simulink model "gyroscope_sym"  (R2025b)
settings: Solver=VariableStepAuto  StartTime=0.0  StopTime=10.0  RelTol=1e-3
values from neighbouring files (symbols this model uses):
  A_bn0 = eye(3)    [gyroscope.m]
  D_bias_inst = 0.3/3600    (= 8.33333333333e-05)    [gyroscope.m]
  D_RW = RRW/sqrt(3600)    [gyroscope.m]
  D_wn = D_ARW/sqrt(3600)    [gyroscope.m]
  I = diag([Ix Iy Iz])    [gyroscope.m]
  O = [1,      eps_xy, eps_xz ... (first row only)    [gyroscope.m]
  run_run_bias = 4/3600    (= 0.00111111111111)    [gyroscope.m]
  SFE = 500*1e-6    (= 0.0005)    [gyroscope.m]
  SFN = 15*1e-6    (= 1.5e-05)    [gyroscope.m]
  static_temp_bias = 9/3600    (= 0.0025)    [gyroscope.m]
  theta_eps = [0,            -theta_eps_z,  theta_eps_y ... (first row only)    [gyroscope.m]
  Ts = 1/update_rate    (= 0.01)    [gyroscope.m]
  w0 = [1e-6; 1e-6; n]    [gyroscope.m]
undefined symbols (not defined in the file or in its folder): DiscIntNeverNeededParam
libraries: matrix_library x4, simulink_extras x1
settings Model: Creator=filip  LastModifiedBy=nicol

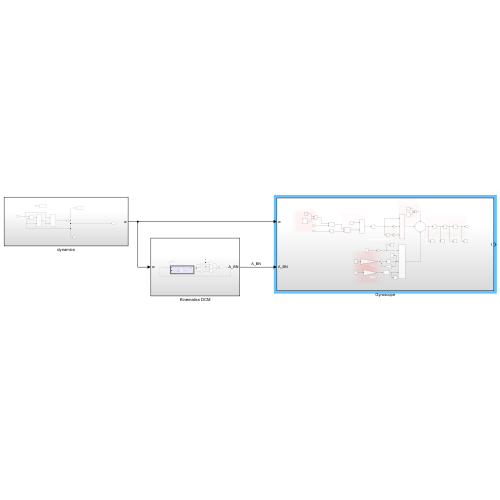
[thumbnail: Simulink's stored preview of the top-level diagram]
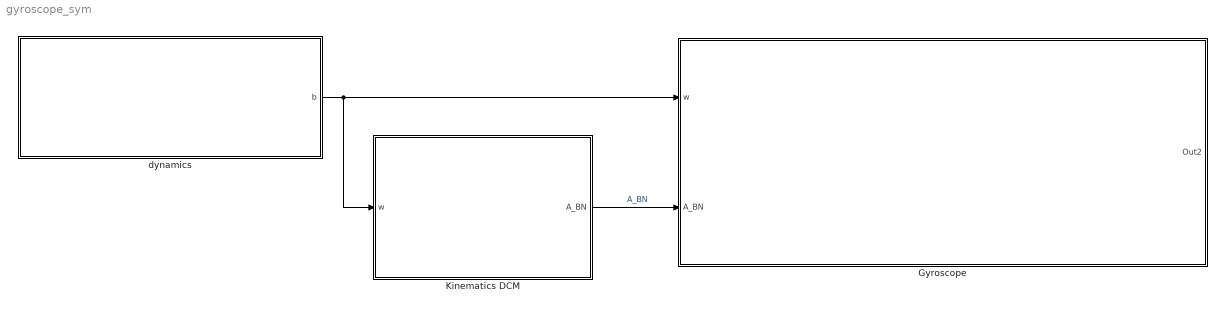
== system gyroscope_sym ==
  Gyroscope : Subsystem
  Kinematics DCM : Subsystem
  dynamics : Subsystem
  wires:
  dynamics/1(b) -> Gyroscope/1(w), Kinematics DCM/1(w)
  Kinematics DCM/1(A_BN) -> Gyroscope/2(A_BN)  "A_BN"

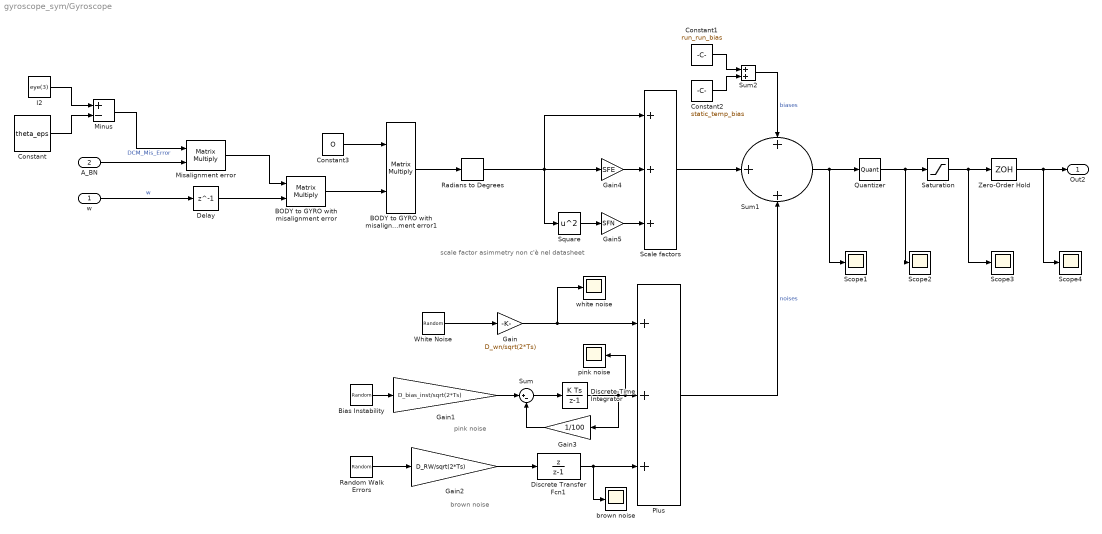
== system gyroscope_sym/Gyroscope ==
  note: scale factor asimmetry non c'è nel datasheet
  note: pink noise
  note: brown noise
  w : Inport
  A_BN : Inport  Port=2
  " White Noise" : RandomNumber  SampleTime=0.1
  BODY to GYRO with misalignment error : Product  Multiplication=Matrix(*)
  BODY to GYRO with misalignment error1 : Product  Multiplication=Matrix(*)
  Bias Instability : RandomNumber  SampleTime=0.1
  Constant : Constant  Value=theta_eps
  Constant1 : Constant  Value=run_run_bias
  Constant2 : Constant  Value=static_temp_bias
  Constant3 : Constant  Value=O
  Delay : Delay  DelayLength=1
  Discrete Transfer Fcn1 : DiscreteTransferFcn  Numerator=[1 0]  Denominator=[1 -1]
  Discrete-Time Integrator : DiscreteIntegrator  ICPrevOutput=DiscIntNeverNeededParam  ICPrevScaledInput=DiscIntNeverNeededParam
  Gain : Gain  Gain=D_wn/sqrt(2*Ts)
  Gain1 : Gain  Gain=D_bias_inst/sqrt(2*Ts)
  Gain2 : Gain  Gain=D_RW/sqrt(2*Ts)
  Gain3 : Gain  Gain=1/100
  Gain4 : Gain  Gain=SFE
  Gain5 : Gain  Gain=SFN
  I2 : Constant  Value=eye(3)
  Minus : Sum  Inputs=+-
  Misalignment error : Product  Multiplication=Matrix(*)
  Plus : Sum  Inputs=+++
  Quantizer : Quantizer  QuantizationInterval=LSB
  Radians to Degrees : simulink_extras/Transformations/Radians to Degrees
  Random Walk Errors : RandomNumber  SampleTime=0.1
  Saturation : Saturate  UpperLimit=20  LowerLimit=-20
  Scale factors : Sum  Inputs=+++
  Scope{1..4} (4 alike) : Scope
      Scope1 settings: ActiveDisplayYMinimum=-0.032120647567430112  ActiveDisplayYMaximum=0.096644162809020939  DataLoggingVariableName=ScopeData2
      Scope2 settings: ActiveDisplayYMinimum=-1  ActiveDisplayYMaximum=1  DataLoggingVariableName=ScopeData3
      Scope3 settings: ActiveDisplayYMinimum=-1  ActiveDisplayYMaximum=1  DataLoggingVariableName=ScopeData4
      Scope4 settings: ActiveDisplayYMinimum=-0.032120647471039  ActiveDisplayYMaximum=0.096644162883216228  DataLoggingVariableName=ScopeData5
  Square : Math  Operator=square
  Sum : Sum  Inputs=|+-
  Sum1 : Sum  Inputs=+++
  Sum2 : Sum
  Zero-Order Hold : ZeroOrderHold  SampleTime=Ts
  brown noise : Scope
      settings: ActiveDisplayYMinimum=-0.025691906984189852  ActiveDisplayYMaximum=0.0025755592198982418  DataLoggingVariableName=ScopeData10
  pink noise : Scope
      settings: ActiveDisplayYMinimum=-0.013777619312277414  ActiveDisplayYMaximum=0.014220901201123974  DataLoggingVariableName=ScopeData9
  white noise : Scope
      settings: ActiveDisplayYMinimum=-0.0017013348354620785  ActiveDisplayYMaximum=0.001720930099973718  DataLoggingVariableName=ScopeData8
  Out2 : Outport
  wires:
  Sum1/1 -> Scope1/1, Quantizer/1
  Gain1/1 -> Sum/1
  A_BN/1 -> Misalignment error/2
  Discrete-Time Integrator/1 -> pink noise/1, Plus/2, Gain3/1
  Gain/1 -> white noise/1, Plus/1
  Plus/1 -> Sum1/3  "noises"
  Random Walk Errors/1 -> Gain2/1
  Constant1/1 -> Sum2/1
  Bias Instability/1 -> Gain1/1
  Discrete Transfer Fcn1/1 -> Plus/3, brown noise/1
  Sum/1 -> Discrete-Time Integrator/1
  I2/1 -> Minus/1
  " White Noise"/1 -> Gain/1
  w/1 -> Delay/1  "w"
  Quantizer/1 -> Scope2/1, Saturation/1
  Minus/1 -> Misalignment error/1  "DCM_Mis_Error"
  Misalignment error/1 -> BODY to GYRO with misalignment error/1
  Saturation/1 -> Scope3/1, Zero-Order Hold/1
  Gain3/1 -> Sum/2
  Zero-Order Hold/1 -> Scope4/1, Out2/1
  Gain2/1 -> Discrete Transfer Fcn1/1
  Delay/1 -> BODY to GYRO with misalignment error/2
  BODY to GYRO with misalignment error/1 -> BODY to GYRO with misalignment error1/2
  Radians to Degrees/1 -> Scale factors/1, Gain4/1, Square/1
  Gain4/1 -> Scale factors/2
  Scale factors/1 -> Sum1/2
  Constant2/1 -> Sum2/2
  Sum2/1 -> Sum1/1  "biases"
  Constant/1 -> Minus/2
  Square/1 -> Gain5/1
  Gain5/1 -> Scale factors/3
  Constant3/1 -> BODY to GYRO with misalignment error1/1
  BODY to GYRO with misalignment error1/1 -> Radians to Degrees/1

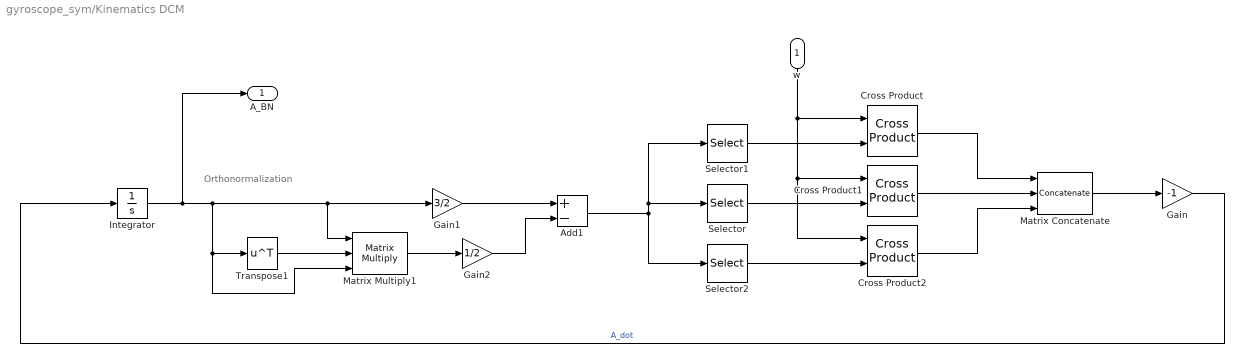
== system gyroscope_sym/Kinematics DCM ==
  note: Orthonormalization
  w : Inport
  Add1 : Sum  Inputs=+-
  Cross Product : matrix_library/Cross Product
  Cross Product1 : matrix_library/Cross Product
  Cross Product2 : matrix_library/Cross Product
  Gain : Gain  Gain=-1
  Gain1 : Gain  Gain=3/2
  Gain2 : Gain  Gain=1/2
  Integrator : Integrator  InitialCondition=A_bn0
  Matrix Concatenate : Concatenate  NumInputs=3  Mode=Multidimensional array  ConcatenateDimension=2
  Matrix Multiply1 : Product  Inputs=3  Multiplication=Matrix(*)
  Selector : Selector  NumberOfDimensions=2  InputPortWidth=3  IndexOptions=Select all,Index vector (dialog)  Indices=[1 3],2  OutputSizes=1,1
  Selector1 : Selector  NumberOfDimensions=2  InputPortWidth=3  IndexOptions=Select all,Index vector (dialog)  Indices=[1 3],1  OutputSizes=1,1
  Selector2 : Selector  NumberOfDimensions=2  InputPortWidth=3  IndexOptions=Select all,Index vector (dialog)  Indices=[1 3],3  OutputSizes=1,1
  Transpose1 : Math  Operator=transpose
  A_BN : Outport
  wires:
  Transpose1/1 -> Matrix Multiply1/2
  w/1 -> Cross Product/1, Cross Product1/1, Cross Product2/1
  Gain/1 -> Integrator/1  "A_dot"
  Gain2/1 -> Add1/2
  Selector/1 -> Cross Product1/2
  Cross Product2/1 -> Matrix Concatenate/3
  Cross Product1/1 -> Matrix Concatenate/2
  Matrix Concatenate/1 -> Gain/1
  Selector1/1 -> Cross Product/2
  Add1/1 -> Selector/1, Selector1/1, Selector2/1
  Matrix Multiply1/1 -> Gain2/1
  Selector2/1 -> Cross Product2/2
  Integrator/1 -> A_BN/1, Transpose1/1, Matrix Multiply1/3, Gain1/1, Matrix Multiply1/1
  Cross Product/1 -> Matrix Concatenate/1
  Gain1/1 -> Add1/1

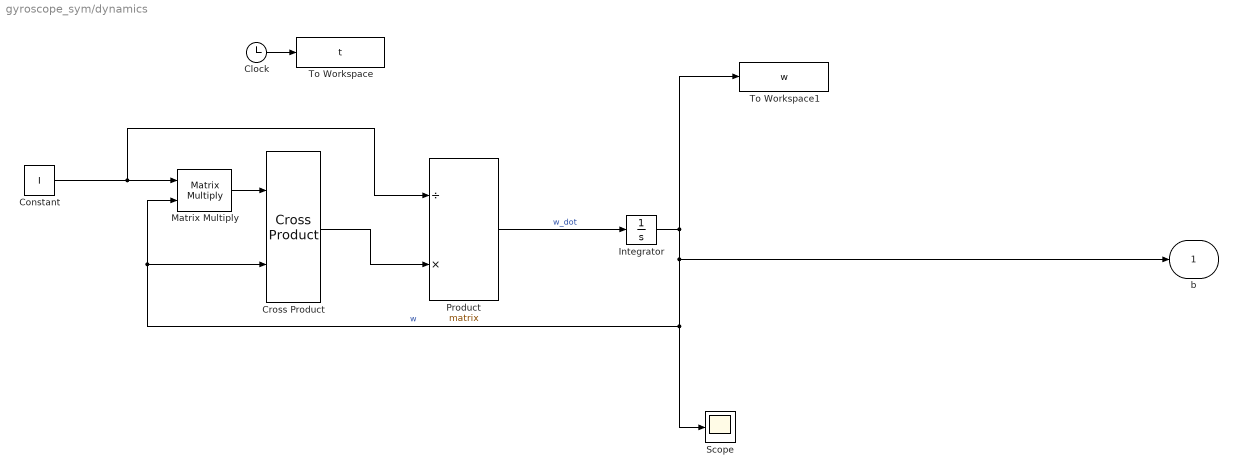
== system gyroscope_sym/dynamics ==
  Clock : Clock
  Constant : Constant  Value=I
  Cross Product : matrix_library/Cross Product
  Integrator : Integrator  InitialCondition=w0
  Matrix Multiply : Product  Multiplication=Matrix(*)
  Product : Product  Inputs=/*  Multiplication=Matrix(*)
  Scope : Scope
      settings: ActiveDisplayYMinimum=-0.00024208345445345938  ActiveDisplayYMaximum=0.0012415118098727709
  To Workspace : ToWorkspace  VariableName=t  SampleTime=-1
  To Workspace1 : ToWorkspace  VariableName=w  SampleTime=-1
  b : Outport
  wires:
  Clock/1 -> To Workspace/1
  Integrator/1 -> b/1, Scope/1, Matrix Multiply/2, Cross Product/2, To Workspace1/1  "w"
  Constant/1 -> Product/1, Matrix Multiply/1
  Cross Product/1 -> Product/2
  Product/1 -> Integrator/1  "w_dot"
  Matrix Multiply/1 -> Cross Product/1
